simulink model "HYD21"  (R2018b)
settings: configuration reference "Test_Config" (kept outside this file)
undefined symbols (not defined in the file): EDP_PRESS, ENG_SPD_RPM, FALSE, HI_PRES_THRE, LO_PRES_THRS, TRUE
libraries: simulink x16
(part 1 of 2)
settings Model: DataDictionary=ARJ21_Dic.sldd  Creator=maoqiang.huang  LastModifiedBy=IT

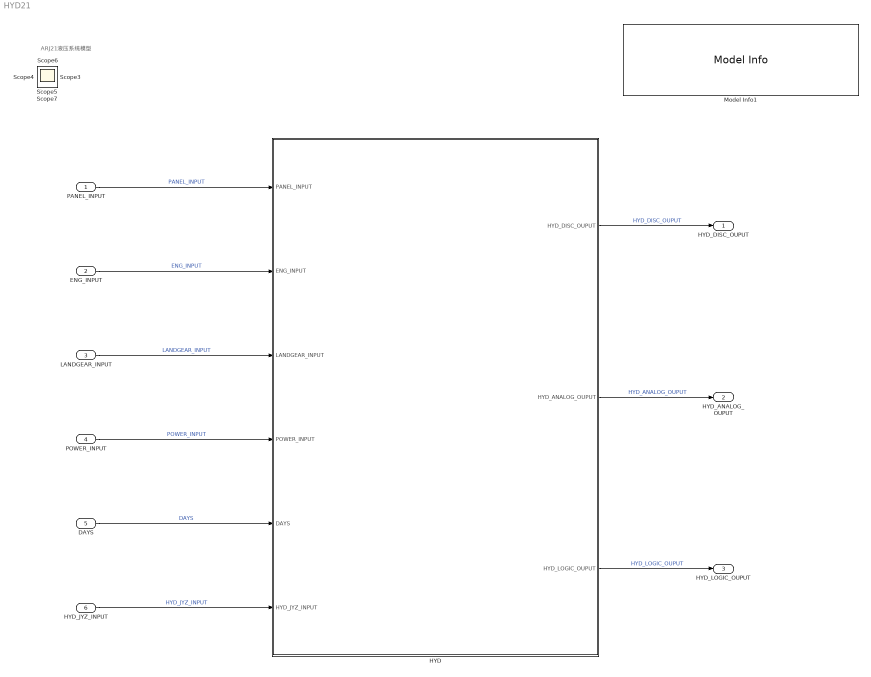
== system HYD21 ==
  note: ARJ21液压系统模型
  PANEL_INPUT : Inport  OutDataTypeStr=Bus: HYD_PANEL_INPUT
  ENG_INPUT : Inport  Port=2  OutDataTypeStr=Bus: HYD_ENG_INPUT
  LANDGEAR_INPUT : Inport  Port=3  OutDataTypeStr=Bus: HYD_LANDGEAR_INPUT
  POWER_INPUT : Inport  Port=4  OutDataTypeStr=Bus: HYD_POWER_INPUT
  DAYS : Inport  Port=5  OutDataTypeStr=uint32
  HYD_JYZ_INPUT : Inport  Port=6  OutDataTypeStr=Bus: HYD_JYZ_INPUT
  HYD : Subsystem
  Model Info1 : simulink/Model-Wide Utilities/Model Info  Frame=on  DisplayStringWithTags=|  HorizontalTextAlignment=Left  LeftAlignmentValue=0.02
      | 创建者：%<Creator>
      | 修改日期：%<ModifiedDate>
      | 模型版本：%<ModelVersion>
  HYD_DISC_OUPUT : Outport  OutDataTypeStr=Bus: HYD_DISC_OUTPUT
  HYD_ANALOG_OUPUT : Outport  Port=2  OutDataTypeStr=Bus: HYD_ANALOG_OUPUT
  HYD_LOGIC_OUPUT : Outport  Port=3  OutDataTypeStr=Bus: HYD_LOGIC_OUPUT
  Scope{,1..7} (8 alike) : Scope
  wires:
  HYD/1(HYD_DISC_OUPUT) -> HYD_DISC_OUPUT/1  "HYD_DISC_OUPUT"
  HYD/2(HYD_ANALOG_OUPUT) -> HYD_ANALOG_OUPUT/1  "HYD_ANALOG_OUPUT"
  PANEL_INPUT/1 -> HYD/1(PANEL_INPUT)  "PANEL_INPUT"
  POWER_INPUT/1 -> HYD/4(POWER_INPUT)  "POWER_INPUT"
  ENG_INPUT/1 -> HYD/2(ENG_INPUT)  "ENG_INPUT"
  LANDGEAR_INPUT/1 -> HYD/3(LANDGEAR_INPUT)  "LANDGEAR_INPUT"
  HYD/3(HYD_LOGIC_OUPUT) -> HYD_LOGIC_OUPUT/1  "HYD_LOGIC_OUPUT"
  DAYS/1 -> HYD/5(DAYS)  "DAYS"
  HYD_JYZ_INPUT/1 -> HYD/6(HYD_JYZ_INPUT)  "HYD_JYZ_INPUT"

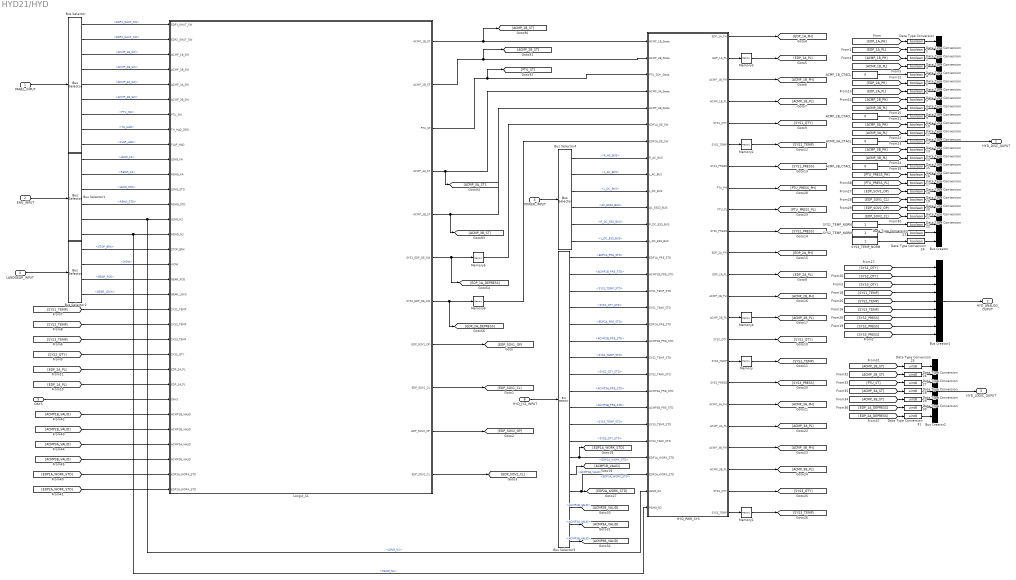
== system HYD21/HYD ==
  PANEL_INPUT : Inport  OutDataTypeStr=Bus: HYD_PANEL_INPUT
  ENG_INPUT : Inport  Port=2  OutDataTypeStr=Bus: HYD_ENG_INPUT
  LANDGEAR_INPUT : Inport  Port=3  OutDataTypeStr=Bus: HYD_LANDGEAR_INPUT
  POWER_INPUT : Inport  Port=4  OutDataTypeStr=Bus: HYD_POWER_INPUT
  DAYS : Inport  Port=5  OutDataTypeStr=uint32
  HYD_JYZ_INPUT : Inport  Port=6  OutDataTypeStr=Bus: HYD_JYZ_INPUT
  ACMP_1B_CTACL : Constant  Value=0
  ACMP_2B_CTACL : Constant  Value=0
  ACMP_3A_CTACL : Constant  Value=0
  ACMP_3B_CTACL : Constant  Value=0
  Bus Creator : BusCreator  Inputs=25  OutDataTypeStr=Bus: HYD_DISC_OUTPUT
  Bus Creator1 : BusCreator  Inputs=9
  Bus Creator2 : BusCreator  Inputs=7
  Bus Selector : BusSelector  OutputSignals=EDP1_SHUT_SW,EDP2_SHUT_SW,ACMP_1B_SW,ACMP_2B_SW,ACMP_3A_SW,ACMP_3B_SW,PTU_SW,TH_HAD,FLAP_HAD
  Bus Selector1 : BusSelector  OutputSignals=LENG_FA,RENG_FA,LENG_STD,RENG_STD,LENG_N2,RENG_N2
  Bus Selector2 : BusSelector  OutputSignals=STOP_BRK,WOW,GEAR_POS,GEAR_LOCK
  Bus Selector3 : BusSelector  OutputSignals=EDP1A_PRE_STD,ACMP1B_PRE_STD,SYS1_TEMP_STD,SYS1_QTY_STD,EDP2A_PRE_STD,ACMP2B_PRE_STD,SYS2_TEMP_STD,SYS2_QTY_STD,ACMP3A_PRE_STD,ACMP3B_PRE_STD,SYS3_TEMP_STD,SYS3_QTY_STD,EDP1A_WORK_STD,ACMP1B_VALID,EDP2A_WORK_STD,ACMP2B_VALID,ACMP3A_VALID,ACMP3B_VALID
  Bus Selector4 : BusSelector  OutputSignals=R_AC_BUS,L_AC_BUS,L_DC_BUS,AC_ESS3_BUS,R_DC_ESS_BUS,L_DC_ESS_BUS
  Data Type Conversion{,1..24} (25 alike) : DataTypeConversion  OutDataTypeStr=boolean
  Data Type Conversion{25..31} (7 alike) : DataTypeConversion  OutDataTypeStr=uint8
  HYD_PWR_SYS : Subsystem
  Locgic_CL : Stateflow chart  TreatAsAtomicUnit=on
  Memory{,1..6} (7 alike) : Memory
  SYS1_TEMP_NORM : Constant
  SYS2_TEMP_NORM : Constant
  SYS3_TEMP_NORM : Constant
  HYD_DISC_OUPUT : Outport  OutDataTypeStr=Bus: HYD_DISC_OUTPUT
  HYD_ANALOG_OUPUT : Outport  Port=2  OutDataTypeStr=Bus: HYD_ANALOG_OUPUT
  HYD_LOGIC_OUPUT : Outport  Port=3  OutDataTypeStr=Bus: HYD_LOGIC_OUPUT
  wires:
  HYD_PWR_SYS/7(SYS1_PRESS) -> [SYS1_PRESS]
  HYD_PWR_SYS/3(ACMP_1B_PH) -> [ACMP_1B_PH]
  Bus Selector1/2 -> Locgic_CL/11(RENG_FA)  "<RENG_FA>"
  [SYS3_TEMP] -> Locgic_CL/22(SYS3_TEMP)
  HYD_PWR_SYS/10(SYS2_PRESS) -> [SYS2_PRESS]
  HYD_PWR_SYS/14(ACMP_2B_PL) -> Memory4/1
  PANEL_INPUT/1 -> Bus Selector/1
  ENG_INPUT/1 -> Bus Selector1/1
  LANDGEAR_INPUT/1 -> Bus Selector2/1
  HYD_PWR_SYS/12(EDP_2A_PL) -> [EDP_2A_PL]
  HYD_PWR_SYS/13(ACMP_2B_PH) -> [ACMP_2B_PH]
  HYD_PWR_SYS/19(ACMP_3A_PL) -> [ACMP_3A_PL]
  Locgic_CL/1(ACMP_1B_ST) -> [ACMP_1B_ST], HYD_PWR_SYS/1(ACMP_1B_State)
  HYD_PWR_SYS/2(EDP_1A_PL) -> Memory3/1
  [EDP_2A_PL] -> Locgic_CL/24(EDP_2A_PL)
  [SYS2_TEMP] -> Locgic_CL/21(SYS2_TEMP)
  Bus Selector1/6 -> HYD_PWR_SYS/29(RENG_N2), Locgic_CL/15(RENG_N2)  "<RENG_N2>"
  HYD_PWR_SYS/20(ACMP_3B_PH) -> [ACMP_3B_PH]
  HYD_PWR_SYS/22(SYS3_QTY) -> [SYS3_QTY]
  Memory6/1 -> HYD_PWR_SYS/7(EDP2A_DE_SW)
  Bus Selector1/5 -> HYD_PWR_SYS/28(LENG_N2), Locgic_CL/14(LENG_N2)  "<LENG_N2>"
  HYD_PWR_SYS/1(EDP_1A_PH) -> [EDP_1A_PH]
  HYD_PWR_SYS/18(ACMP_3A_PH) -> [ACMP_3A_PH]
  HYD_PWR_SYS/15(SYS2_QTY) -> [SYS2_QTY]
  HYD_PWR_SYS/21(ACMP_3B_PL) -> [ACMP_3B_PL]
  Bus Selector1/3 -> Locgic_CL/12(LENG_STD)  "<LENG_STD>"
  HYD_PWR_SYS/17(SYS3_PRESS) -> [SYS3_PRESS]
  Bus Selector/1 -> Locgic_CL/1(EDP1_SHUT_SW)  "<EDP1_SHUT_SW>"
  Bus Selector/6 -> Locgic_CL/6(ACMP_3B_SW)  "<ACMP_3B_SW>"
  Bus Selector/9 -> Locgic_CL/9(FLAP_HAD)  "<FLAP_HAD>"
  Bus Selector/8 -> Locgic_CL/8(TH_HAD_DEG)  "<TH_HAD>"
  Bus Selector/2 -> Locgic_CL/2(EDP2_SHUT_SW)  "<EDP2_SHUT_SW>"
  Bus Selector/5 -> Locgic_CL/5(ACMP_3A_SW)  "<ACMP_3A_SW>"
  Bus Selector/3 -> Locgic_CL/3(ACMP_1B_SW)  "<ACMP_1B_SW>"
  Bus Selector/7 -> Locgic_CL/7(PTU_SW)  "<PTU_SW>"
  Bus Selector/4 -> Locgic_CL/4(ACMP_2B_SW)  "<ACMP_2B_SW>"
  [SYS2_QTY] -> Locgic_CL/23(SYS2_QTY)
  Bus Selector2/1 -> Locgic_CL/16(STOP_BRK)  "<STOP_BRK>"
  Bus Selector2/2 -> Locgic_CL/17(WOW)  "<WOW>"
  Bus Selector2/3 -> Locgic_CL/18(GEAR_POS)  "<GEAR_POS>"
  Bus Selector2/4 -> Locgic_CL/19(GEAR_LOCK)  "<GEAR_LOCK>"
  POWER_INPUT/1 -> Bus Selector4/1
  [SYS1_TEMP] -> Locgic_CL/20(SYS1_TEMP)
  Locgic_CL/8(EDP_SOV1_OP) -> [EDP_SOV1_OP]
  Data Type Conversion11/1 -> Bus Creator/12
  Data Type Conversion12/1 -> Bus Creator/13
  Data Type Conversion3/1 -> Bus Creator/4
  [EDP_1A_PH] -> Data Type Conversion/1
  ACMP_1B_CTACL/1 -> Data Type Conversion4/1
  [EDP_SOV2_OP] -> Data Type Conversion20/1
  Data Type Conversion1/1 -> Bus Creator/2
  Data Type Conversion7/1 -> Bus Creator/8
  Data Type Conversion8/1 -> Bus Creator/9
  ACMP_3A_CTACL/1 -> Data Type Conversion12/1
  [ACMP_3B_PL] -> Data Type Conversion14/1
  SYS1_TEMP_NORM/1 -> Data Type Conversion22/1
  Data Type Conversion4/1 -> Bus Creator/5
  Data Type Conversion10/1 -> Bus Creator/11
  Data Type Conversion13/1 -> Bus Creator/14
  Data Type Conversion14/1 -> Bus Creator/15
  [ACMP_2B_PH] -> Data Type Conversion7/1
  [ACMP_3A_PH] -> Data Type Conversion10/1
  [PTU_PRESS_PH] -> Data Type Conversion16/1
  [ACMP_3B_PH] -> Data Type Conversion13/1
  ACMP_3B_CTACL/1 -> Data Type Conversion15/1
  [EDP_SOV2_CL] -> Data Type Conversion21/1
  Data Type Conversion2/1 -> Bus Creator/3
  Data Type Conversion5/1 -> Bus Creator/6
  [EDP_1A_PL] -> Data Type Conversion1/1
  ACMP_2B_CTACL/1 -> Data Type Conversion9/1
  [EDP_2A_PL] -> Data Type Conversion6/1
  [ACMP_1B_PL] -> Data Type Conversion3/1
  [EDP_2A_PH] -> Data Type Conversion5/1
  [ACMP_2B_PL] -> Data Type Conversion8/1
  [ACMP_3A_PL] -> Data Type Conversion11/1
  [EDP_SOV1_CL] -> Data Type Conversion19/1
  SYS3_TEMP_NORM/1 -> Data Type Conversion24/1
  [EDP_SOV1_OP] -> Data Type Conversion18/1
  SYS2_TEMP_NORM/1 -> Data Type Conversion23/1
  Data Type Conversion/1 -> Bus Creator/1
  [ACMP_1B_PH] -> Data Type Conversion2/1
  Data Type Conversion6/1 -> Bus Creator/7
  Data Type Conversion9/1 -> Bus Creator/10
  Data Type Conversion17/1 -> Bus Creator/18
  [SYS2_QTY] -> Bus Creator1/2
  [SYS3_QTY] -> Bus Creator1/3
  Data Type Conversion21/1 -> Bus Creator/22
  [SYS1_TEMP] -> Bus Creator1/4
  [SYS2_PRESS] -> Bus Creator1/8
  [SYS3_PRESS] -> Bus Creator1/9
  Data Type Conversion24/1 -> Bus Creator/25
  Data Type Conversion23/1 -> Bus Creator/24
  [SYS3_TEMP] -> Bus Creator1/6
  Data Type Conversion15/1 -> Bus Creator/16
  Data Type Conversion18/1 -> Bus Creator/19
  Data Type Conversion20/1 -> Bus Creator/21
  Data Type Conversion22/1 -> Bus Creator/23
  [SYS2_TEMP] -> Bus Creator1/5
  Data Type Conversion19/1 -> Bus Creator/20
  [SYS1_PRESS] -> Bus Creator1/7
  Data Type Conversion16/1 -> Bus Creator/17
  [SYS1_QTY] -> Bus Creator1/1
  Bus Selector4/3 -> HYD_PWR_SYS/10(L_DC_BUS)  "<L_DC_BUS>"
  Bus Selector4/5 -> HYD_PWR_SYS/12(R_DC_ESS_BUS)  "<R_DC_ESS_BUS>"
  Bus Selector4/1 -> HYD_PWR_SYS/8(R_AC_BUS)  "<R_AC_BUS>"
  Bus Selector4/6 -> HYD_PWR_SYS/13(L_DC_ESS_BUS)  "<L_DC_ESS_BUS>"
  Bus Selector4/2 -> HYD_PWR_SYS/9(L_AC_BUS)  "<L_AC_BUS>"
  Bus Selector4/4 -> HYD_PWR_SYS/11(AC_ESS3_BUS)  "<AC_ESS3_BUS>"
  Bus Selector1/4 -> Locgic_CL/13(RENG_STD)  "<RENG_STD>"
  HYD_PWR_SYS/23(SYS3_TEMP) -> Memory1/1
  HYD_PWR_SYS/11(EDP_2A_PH) -> [EDP_2A_PH]
  Memory/1 -> [SYS2_TEMP]
  Bus Selector1/1 -> Locgic_CL/10(LENG_FA)  "<LENG_FA>"
  HYD_PWR_SYS/6(SYS1_TEMP) -> Memory2/1
  [EDP_1A_PL] -> Locgic_CL/25(EDP_1A_PL)
  HYD_PWR_SYS/16(SYS2_TEMP) -> Memory/1
  HYD_PWR_SYS/5(SYS1_QTY) -> [SYS1_QTY]
  Locgic_CL/11(EDP_SOV2_CL) -> [EDP_SOV2_CL]
  Memory1/1 -> [SYS3_TEMP]
  Memory2/1 -> [SYS1_TEMP]
  Memory3/1 -> [EDP_1A_PL]
  Memory4/1 -> [ACMP_2B_PL]
  Memory5/1 -> HYD_PWR_SYS/6(EDP1A_DE_SW)
  HYD_PWR_SYS/4(ACMP_1B_PL) -> [ACMP_1B_PL]
  DAYS/1 -> Locgic_CL/26(DAYS)
  Locgic_CL/9(EDP_SOV1_CL) -> [EDP_SOV1_CL]
  Locgic_CL/6(SYS1_EDP_DE_SW) -> [EDP_1A_DEPRESS], Memory5/1
  Locgic_CL/7(SYS2_EDP_DE_SW) -> [EDP_2A_DEPRESS], Memory6/1
  Locgic_CL/3(PTU_ST) -> [PTU_ST], HYD_PWR_SYS/3(PTU_SOV_State)
  Locgic_CL/5(ACMP_3B_ST) -> [ACMP_3B_ST], HYD_PWR_SYS/5(ACMP_3B_State)
  Locgic_CL/4(ACMP_3A_ST) -> [ACMP_3A_ST], HYD_PWR_SYS/4(ACMP_3A_State)
  Locgic_CL/10(EDP_SOV2_OP) -> [EDP_SOV2_OP]
  Locgic_CL/2(ACMP_2B_ST) -> [ACMP_2B_ST], HYD_PWR_SYS/2(ACMP_2B_State)
  Bus Creator1/1 -> HYD_ANALOG_OUPUT/1
  Bus Creator/1 -> HYD_DISC_OUPUT/1
  HYD_PWR_SYS/8(PTU_PH) -> [PTU_PRESS_PH]
  HYD_PWR_SYS/9(PTU_PL) -> [PTU_PRESS_PL]
  [PTU_PRESS_PL] -> Data Type Conversion17/1
  Bus Creator2/1 -> HYD_LOGIC_OUPUT/1
  [ACMP_2B_ST] -> Data Type Conversion26/1
  [ACMP_3B_ST] -> Data Type Conversion29/1
  [ACMP_3A_ST] -> Data Type Conversion28/1
  [PTU_ST] -> Data Type Conversion27/1
  [ACMP_1B_ST] -> Data Type Conversion25/1
  [EDP_2A_DEPRESS] -> Data Type Conversion31/1
  [EDP_1A_DEPRESS] -> Data Type Conversion30/1
  Data Type Conversion25/1 -> Bus Creator2/1
  Data Type Conversion26/1 -> Bus Creator2/2
  Data Type Conversion27/1 -> Bus Creator2/3
  Data Type Conversion28/1 -> Bus Creator2/4
  Data Type Conversion29/1 -> Bus Creator2/5
  Data Type Conversion30/1 -> Bus Creator2/6
  Data Type Conversion31/1 -> Bus Creator2/7
  HYD_JYZ_INPUT/1 -> Bus Selector3/1
  Bus Selector3/1 -> HYD_PWR_SYS/14(EDP1A_PRE_STD)  "<EDP1A_PRE_STD>"
  Bus Selector3/13 -> HYD_PWR_SYS/26(EDP1A_WORK_STD), [EDP1A_WORK_STD]  "<EDP1A_WORK_STD>"
  Bus Selector3/14 -> [ACMP1B_VALID]  "<ACMP1B_VALID>"
  Bus Selector3/16 -> [ACMP2B_VALID]  "<ACMP2B_VALID>"
  [EDP1A_WORK_STD] -> Locgic_CL/31(EDP1A_WORK_STD)
  [EDP2A_WORK_STD] -> Locgic_CL/32(EDP2A_WORK_STD)
  [ACMP1B_VALID] -> Locgic_CL/27(ACMP1B_VALID)
  [ACMP2B_VALID] -> Locgic_CL/28(ACMP2B_VALID)
  Bus Selector3/17 -> [ACMP3A_VALID]  "<ACMP3A_VALID>"
  Bus Selector3/18 -> [ACMP3B_VALID]  "<ACMP3B_VALID>"
  [ACMP3A_VALID] -> Locgic_CL/29(ACMP3A_VALID)
  [ACMP3B_VALID] -> Locgic_CL/30(ACMP3B_VALID)
  Bus Selector3/2 -> HYD_PWR_SYS/15(ACMP1B_PRE_STD)  "<ACMP1B_PRE_STD>"
  Bus Selector3/3 -> HYD_PWR_SYS/16(SYS1_TEMP_STD)  "<SYS1_TEMP_STD>"
  Bus Selector3/4 -> HYD_PWR_SYS/17(SYS1_TANK_STD)  "<SYS1_QTY_STD>"
  Bus Selector3/5 -> HYD_PWR_SYS/18(EDP2A_PRE_STD)  "<EDP2A_PRE_STD>"
  Bus Selector3/6 -> HYD_PWR_SYS/19(ACMP2B_PRE_STD)  "<ACMP2B_PRE_STD>"
  Bus Selector3/7 -> HYD_PWR_SYS/20(SYS2_TEMP_STD)  "<SYS2_TEMP_STD>"
  Bus Selector3/8 -> HYD_PWR_SYS/21(SYS2_TANK_STD)  "<SYS2_QTY_STD>"
  Bus Selector3/9 -> HYD_PWR_SYS/22(ACMP3A_PRE_STD)  "<ACMP3A_PRE_STD>"
  Bus Selector3/10 -> HYD_PWR_SYS/23(ACMP3B_PRE_STD)  "<ACMP3B_PRE_STD>"
  Bus Selector3/11 -> HYD_PWR_SYS/24(SYS3_TEMP_STD)  "<SYS3_TEMP_STD>"
  Bus Selector3/12 -> HYD_PWR_SYS/25(SYS3_TANK_STD)  "<SYS3_QTY_STD>"
  Bus Selector3/15 -> HYD_PWR_SYS/27(EDP2A_WORK_STD), [EDP2A_WORK_STD]  "<EDP2A_WORK_STD>"

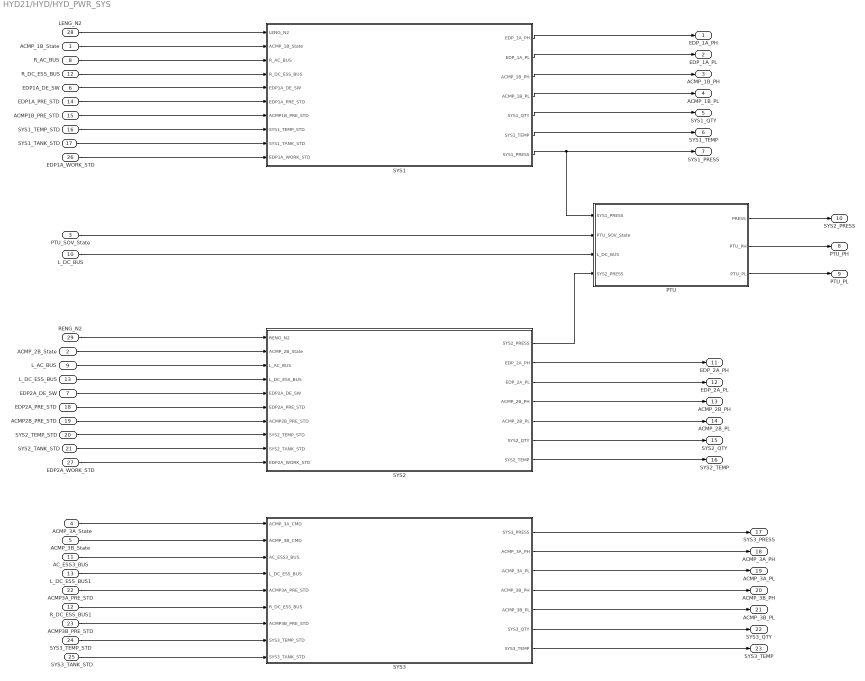
== system HYD21/HYD/HYD_PWR_SYS ==
  ACMP_1B_State : Inport
  ACMP_2B_State : Inport  Port=2
  PTU_SOV_State : Inport  Port=3
  ACMP_3A_State : Inport  Port=4
  ACMP_3B_State : Inport  Port=5
  EDP1A_DE_SW : Inport  Port=6
  EDP2A_DE_SW : Inport  Port=7
  R_AC_BUS : Inport  Port=8
  L_AC_BUS : Inport  Port=9
  L_DC_BUS : Inport  Port=10
  AC_ESS3_BUS : Inport  Port=11
  R_DC_ESS_BUS : Inport  Port=12
  L_DC_ESS_BUS : Inport  Port=13
  EDP1A_PRE_STD : Inport  Port=14
  ACMP1B_PRE_STD : Inport  Port=15
  SYS1_TEMP_STD : Inport  Port=16
  SYS1_TANK_STD : Inport  Port=17
  EDP2A_PRE_STD : Inport  Port=18
  ACMP2B_PRE_STD : Inport  Port=19
  SYS2_TEMP_STD : Inport  Port=20
  SYS2_TANK_STD : Inport  Port=21
  ACMP3A_PRE_STD : Inport  Port=22
  ACMP3B_PRE_STD : Inport  Port=23
  SYS3_TEMP_STD : Inport  Port=24
  SYS3_TANK_STD : Inport  Port=25
  EDP1A_WORK_STD : Inport  Port=26  OutDataTypeStr=uint8
  EDP2A_WORK_STD : Inport  Port=27  OutDataTypeStr=uint8
  LENG_N2 : Inport  Port=28
  RENG_N2 : Inport  Port=29
  L_DC_ESS_BUS1 : InportShadow  Port=13
  PTU : Subsystem
  R_DC_ESS_BUS1 : InportShadow  Port=12
  SYS1 : Subsystem
  SYS2 : Subsystem
  SYS3 : Subsystem
  EDP_1A_PH : Outport
  EDP_1A_PL : Outport  Port=2
  ACMP_1B_PH : Outport  Port=3
  ACMP_1B_PL : Outport  Port=4
  SYS1_QTY : Outport  Port=5
  SYS1_TEMP : Outport  Port=6
  SYS1_PRESS : Outport  Port=7
  PTU_PH : Outport  Port=8
  PTU_PL : Outport  Port=9
  SYS2_PRESS : Outport  Port=10
  EDP_2A_PH : Outport  Port=11
  EDP_2A_PL : Outport  Port=12
  ACMP_2B_PH : Outport  Port=13
  ACMP_2B_PL : Outport  Port=14
  SYS2_QTY : Outport  Port=15
  SYS2_TEMP : Outport  Port=16
  SYS3_PRESS : Outport  Port=17
  ACMP_3A_PH : Outport  Port=18
  ACMP_3A_PL : Outport  Port=19
  ACMP_3B_PH : Outport  Port=20
  ACMP_3B_PL : Outport  Port=21
  SYS3_QTY : Outport  Port=22
  SYS3_TEMP : Outport  Port=23
  wires:
  SYS1/6(SYS1_TEMP) -> SYS1_TEMP/1
  SYS1/3(ACMP_1B_PH) -> ACMP_1B_PH/1
  SYS2/4(ACMP_2B_PH) -> ACMP_2B_PH/1
  SYS2/3(EDP_2A_PL) -> EDP_2A_PL/1
  SYS1/1(EDP_1A_PH) -> EDP_1A_PH/1
  SYS1/2(EDP_1A_PL) -> EDP_1A_PL/1
  SYS1/4(ACMP_1B_PL) -> ACMP_1B_PL/1
  SYS1/5(SYS1_QTY) -> SYS1_QTY/1
  SYS2/2(EDP_2A_PH) -> EDP_2A_PH/1
  SYS2/7(SYS2_TEMP) -> SYS2_TEMP/1
  SYS3/1(SYS3_PRESS) -> SYS3_PRESS/1
  SYS3/7(SYS3_TEMP) -> SYS3_TEMP/1
  SYS2/5(ACMP_2B_PL) -> ACMP_2B_PL/1
  SYS3/4(ACMP_3B_PH) -> ACMP_3B_PH/1
  SYS3/6(SYS3_QTY) -> SYS3_QTY/1
  SYS3/2(ACMP_3A_PH) -> ACMP_3A_PH/1
  SYS2/6(SYS2_QTY) -> SYS2_QTY/1
  SYS3/3(ACMP_3A_PL) -> ACMP_3A_PL/1
  SYS3/5(ACMP_3B_PL) -> ACMP_3B_PL/1
  SYS1/7(SYS1_PRESS) -> SYS1_PRESS/1, PTU/1(SYS1_PRESS)
  LENG_N2/1 -> SYS1/1(LENG_N2)
  ACMP_1B_State/1 -> SYS1/2(ACMP_1B_State)
  EDP1A_DE_SW/1 -> SYS1/5(EDP1A_DE_SW)
  EDP1A_PRE_STD/1 -> SYS1/6(EDP1A_PRE_STD)
  ACMP1B_PRE_STD/1 -> SYS1/7(ACMP1B_PRE_STD)
  SYS1_TEMP_STD/1 -> SYS1/8(SYS1_TEMP_STD)
  SYS1_TANK_STD/1 -> SYS1/9(SYS1_TANK_STD)
  SYS2/1(SYS2_PRESS) -> PTU/4(SYS2_PRESS)
  PTU_SOV_State/1 -> PTU/2(PTU_SOV_State)
  PTU/1(PRESS) -> SYS2_PRESS/1
  L_DC_BUS/1 -> PTU/3(L_DC_BUS)
  ACMP_2B_State/1 -> SYS2/2(ACMP_2B_State)
  RENG_N2/1 -> SYS2/1(RENG_N2)
  L_AC_BUS/1 -> SYS2/3(L_AC_BUS)
  L_DC_ESS_BUS/1 -> SYS2/4(L_DC_ESS_BUS)
  EDP2A_DE_SW/1 -> SYS2/5(EDP2A_DE_SW)
  EDP2A_PRE_STD/1 -> SYS2/6(EDP2A_PRE_STD)
  ACMP2B_PRE_STD/1 -> SYS2/7(ACMP2B_PRE_STD)
  SYS2_TEMP_STD/1 -> SYS2/8(SYS2_TEMP_STD)
  SYS2_TANK_STD/1 -> SYS2/9(SYS2_TANK_STD)
  ACMP_3A_State/1 -> SYS3/1(ACMP_3A_CMD)
  ACMP_3B_State/1 -> SYS3/2(ACMP_3B_CMD)
  L_DC_ESS_BUS1/1 -> SYS3/4(L_DC_ESS_BUS)
  R_DC_ESS_BUS1/1 -> SYS3/6(R_DC_ESS_BUS)
  ACMP3B_PRE_STD/1 -> SYS3/7(ACMP3B_PRE_STD)
  AC_ESS3_BUS/1 -> SYS3/3(AC_ESS3_BUS)
  SYS3_TEMP_STD/1 -> SYS3/8(SYS3_TEMP_STD)
  SYS3_TANK_STD/1 -> SYS3/9(SYS3_TANK_STD)
  ACMP3A_PRE_STD/1 -> SYS3/5(ACMP3A_PRE_STD)
  R_DC_ESS_BUS/1 -> SYS1/4(R_DC_ESS_BUS)
  R_AC_BUS/1 -> SYS1/3(R_AC_BUS)
  PTU/2(PTU_PH) -> PTU_PH/1
  PTU/3(PTU_PL) -> PTU_PL/1
  EDP1A_WORK_STD/1 -> SYS1/10(EDP1A_WORK_STD)
  EDP2A_WORK_STD/1 -> SYS2/10(EDP2A_WORK_STD)

== system HYD21/HYD/HYD_PWR_SYS/PTU ==
  SYS1_PRESS : Inport
  PTU_SOV_State : Inport  Port=2
  L_DC_BUS : Inport  Port=3
  SYS2_PRESS : Inport  Port=4
  Compare To Constant : simulink/Logic and Bit Operations/Compare To Constant  relop=<=  const=1800  OutDataTypeStr=boolean
  HYD2_PRESS_State : Terminator
  Logical Operator : Logic  AllPortsSameDT=off  OutDataTypeStr=boolean
  PRE_SWITCH : Subsystem
  Switch1 : Switch  Criteria=u2 > Threshold  Threshold=LO_PRES_THRS
  PRESS : Outport
  PTU_PH : Outport  Port=2
  PTU_PL : Outport  Port=3
  wires:
  Switch1/1 -> PRE_SWITCH/1(PRE), Compare To Constant/1, PRESS/1
  PTU_SOV_State/1 -> Logical Operator/1
  L_DC_BUS/1 -> Logical Operator/2
  Logical Operator/1 -> Switch1/2
  SYS1_PRESS/1 -> Switch1/1
  SYS2_PRESS/1 -> Switch1/3
  Compare To Constant/1 -> HYD2_PRESS_State/1
  PRE_SWITCH/1(PH) -> PTU_PH/1
  PRE_SWITCH/2(PL) -> PTU_PL/1

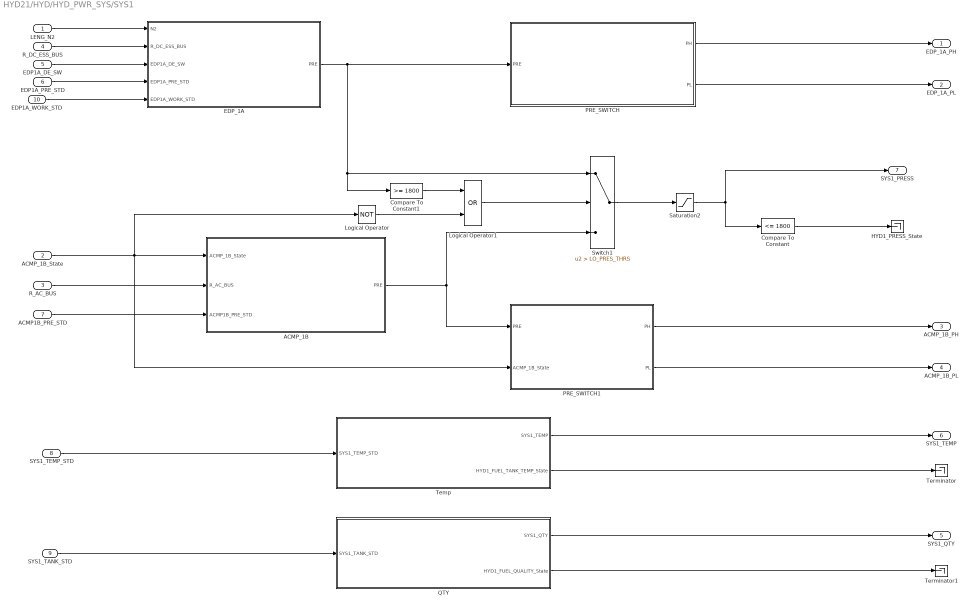
== system HYD21/HYD/HYD_PWR_SYS/SYS1 ==
  LENG_N2 : Inport
  ACMP_1B_State : Inport  Port=2
  R_AC_BUS : Inport  Port=3
  R_DC_ESS_BUS : Inport  Port=4
  EDP1A_DE_SW : Inport  Port=5
  EDP1A_PRE_STD : Inport  Port=6
  ACMP1B_PRE_STD : Inport  Port=7
  SYS1_TEMP_STD : Inport  Port=8
  SYS1_TANK_STD : Inport  Port=9
  EDP1A_WORK_STD : Inport  Port=10  OutDataTypeStr=uint8
  ACMP_1B : Subsystem
  Compare To Constant : simulink/Logic and Bit Operations/Compare To Constant  relop=<=  const=1800  OutDataTypeStr=boolean
  Compare To Constant1 : simulink/Logic and Bit Operations/Compare To Constant  relop=>=  const=1800  OutDataTypeStr=boolean
  EDP_1A : Subsystem
  HYD1_PRESS_State : Terminator
  Logical Operator : Logic  Operator=NOT  AllPortsSameDT=off  OutDataTypeStr=boolean
  Logical Operator1 : Logic  Operator=OR  AllPortsSameDT=off  OutDataTypeStr=boolean
  PRE_SWITCH : Subsystem
  PRE_SWITCH1 : Subsystem
  QTY : Subsystem
  Saturation2 : Saturate  UpperLimit=3000  LowerLimit=0
  Switch1 : Switch  Criteria=u2 > Threshold  Threshold=LO_PRES_THRS
  Temp : Subsystem
  Terminator : Terminator
  Terminator1 : Terminator
  EDP_1A_PH : Outport
  EDP_1A_PL : Outport  Port=2
  ACMP_1B_PH : Outport  Port=3
  ACMP_1B_PL : Outport  Port=4
  SYS1_QTY : Outport  Port=5
  SYS1_TEMP : Outport  Port=6
  SYS1_PRESS : Outport  Port=7
  wires:
  Switch1/1 -> Saturation2/1
  Saturation2/1 -> SYS1_PRESS/1, Compare To Constant/1
  ACMP_1B/1(PRE) -> PRE_SWITCH1/1(PRE), Switch1/3
  PRE_SWITCH/1(PH) -> EDP_1A_PH/1
  PRE_SWITCH/2(PL) -> EDP_1A_PL/1
  EDP_1A/1(PRE) -> Switch1/1, Compare To Constant1/1, PRE_SWITCH/1(PRE)
  PRE_SWITCH1/1(PH) -> ACMP_1B_PH/1
  PRE_SWITCH1/2(PL) -> ACMP_1B_PL/1
  ACMP_1B_State/1 -> PRE_SWITCH1/2(ACMP_1B_State), Logical Operator/1, ACMP_1B/1(ACMP_1B_State)
  Temp/1(SYS1_TEMP) -> SYS1_TEMP/1
  QTY/1(SYS1_QTY) -> SYS1_QTY/1
  LENG_N2/1 -> EDP_1A/1(N2)
  R_DC_ESS_BUS/1 -> EDP_1A/2(R_DC_ESS_BUS)
  EDP1A_DE_SW/1 -> EDP_1A/3(EDP1A_DE_SW)
  EDP1A_PRE_STD/1 -> EDP_1A/4(EDP1A_PRE_STD)
  SYS1_TEMP_STD/1 -> Temp/1(SYS1_TEMP_STD)
  SYS1_TANK_STD/1 -> QTY/1(SYS1_TANK_STD)
  R_AC_BUS/1 -> ACMP_1B/2(R_AC_BUS)
  ACMP1B_PRE_STD/1 -> ACMP_1B/3(ACMP1B_PRE_STD)
  Temp/2("HYD1_FUEL_TANK_TEMP_State ") -> Terminator/1
  QTY/2(HYD1_FUEL_QUALITY_State) -> Terminator1/1
  Compare To Constant/1 -> HYD1_PRESS_State/1
  Logical Operator/1 -> Logical Operator1/2
  Compare To Constant1/1 -> Logical Operator1/1
  Logical Operator1/1 -> Switch1/2
  EDP1A_WORK_STD/1 -> EDP_1A/5(EDP1A_WORK_STD)

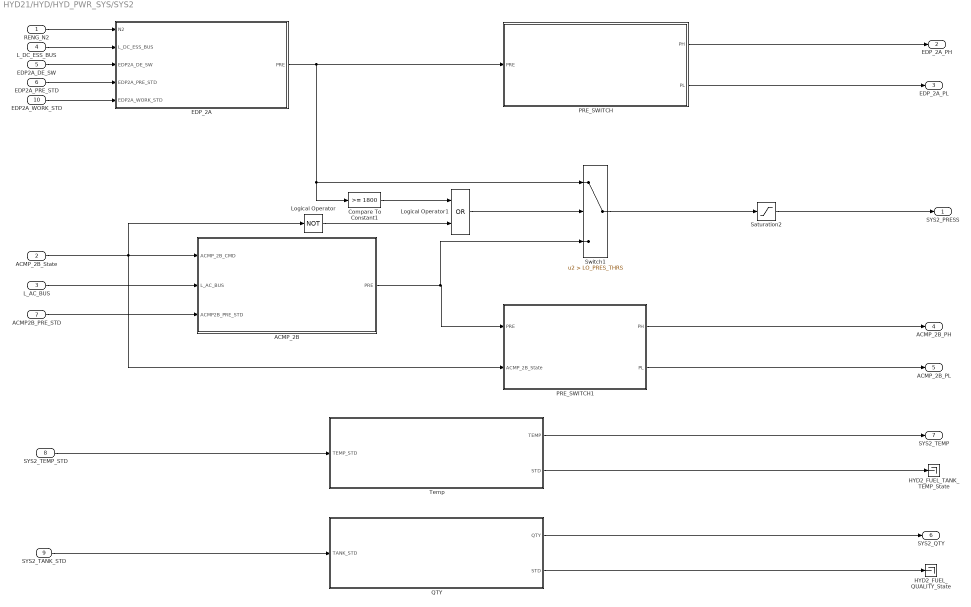
== system HYD21/HYD/HYD_PWR_SYS/SYS2 ==
  RENG_N2 : Inport
  ACMP_2B_State : Inport  Port=2
  L_AC_BUS : Inport  Port=3
  L_DC_ESS_BUS : Inport  Port=4
  EDP2A_DE_SW : Inport  Port=5
  EDP2A_PRE_STD : Inport  Port=6
  ACMP2B_PRE_STD : Inport  Port=7
  SYS2_TEMP_STD : Inport  Port=8
  SYS2_TANK_STD : Inport  Port=9
  EDP2A_WORK_STD : Inport  Port=10  OutDataTypeStr=uint8
  ACMP_2B : Subsystem
  Compare To Constant1 : simulink/Logic and Bit Operations/Compare To Constant  relop=>=  const=1800  OutDataTypeStr=boolean
  EDP_2A : Subsystem
  HYD2_FUEL_QUALITY_State : Terminator
  HYD2_FUEL_TANK_TEMP_State : Terminator
  Logical Operator : Logic  Operator=NOT  AllPortsSameDT=off  OutDataTypeStr=boolean
  Logical Operator1 : Logic  Operator=OR  AllPortsSameDT=off  OutDataTypeStr=boolean
  PRE_SWITCH : Subsystem
  PRE_SWITCH1 : Subsystem
  QTY : Subsystem
  Saturation2 : Saturate  UpperLimit=3000  LowerLimit=0
  Switch1 : Switch  Criteria=u2 > Threshold  Threshold=LO_PRES_THRS
  Temp : Subsystem
  SYS2_PRESS : Outport
  EDP_2A_PH : Outport  Port=2
  EDP_2A_PL : Outport  Port=3
  ACMP_2B_PH : Outport  Port=4
  ACMP_2B_PL : Outport  Port=5
  SYS2_QTY : Outport  Port=6
  SYS2_TEMP : Outport  Port=7
  wires:
  ACMP2B_PRE_STD/1 -> ACMP_2B/3(ACMP2B_PRE_STD)
  L_AC_BUS/1 -> ACMP_2B/2(L_AC_BUS)
  SYS2_TANK_STD/1 -> QTY/1(TANK_STD)
  SYS2_TEMP_STD/1 -> Temp/1(TEMP_STD)
  EDP2A_PRE_STD/1 -> EDP_2A/4(EDP2A_PRE_STD)
  EDP2A_DE_SW/1 -> EDP_2A/3(EDP2A_DE_SW)
  L_DC_ESS_BUS/1 -> EDP_2A/2(L_DC_ESS_BUS)
  RENG_N2/1 -> EDP_2A/1(N2)
  QTY/1(QTY) -> SYS2_QTY/1
  Temp/1(TEMP) -> SYS2_TEMP/1
  ACMP_2B_State/1 -> PRE_SWITCH1/2(ACMP_2B_State), ACMP_2B/1(ACMP_2B_CMD), Logical Operator/1
  PRE_SWITCH1/2(PL) -> ACMP_2B_PL/1
  PRE_SWITCH1/1(PH) -> ACMP_2B_PH/1
  EDP_2A/1(PRE) -> Switch1/1, Compare To Constant1/1, PRE_SWITCH/1(PRE)
  PRE_SWITCH/2(PL) -> EDP_2A_PL/1
  PRE_SWITCH/1(PH) -> EDP_2A_PH/1
  ACMP_2B/1(PRE) -> PRE_SWITCH1/1(PRE), Switch1/3
  Saturation2/1 -> SYS2_PRESS/1
  Switch1/1 -> Saturation2/1
  Temp/2(STD) -> HYD2_FUEL_TANK_TEMP_State/1
  QTY/2(STD) -> HYD2_FUEL_QUALITY_State/1
  Compare To Constant1/1 -> Logical Operator1/1
  Logical Operator/1 -> Logical Operator1/2
  Logical Operator1/1 -> Switch1/2
  EDP2A_WORK_STD/1 -> EDP_2A/5(EDP2A_WORK_STD)

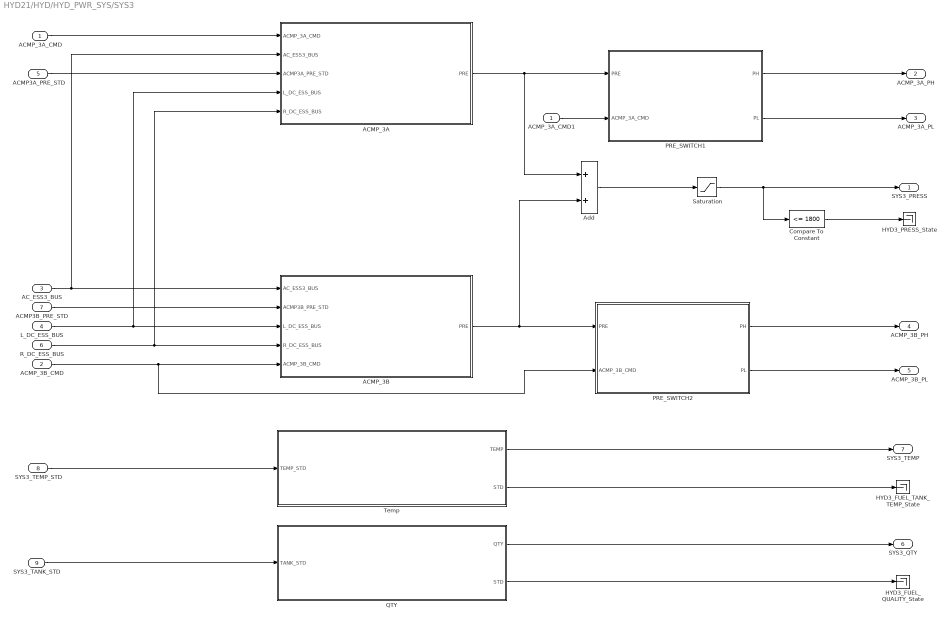
== system HYD21/HYD/HYD_PWR_SYS/SYS3 ==
  ACMP_3A_CMD : Inport
  ACMP_3B_CMD : Inport  Port=2
  AC_ESS3_BUS : Inport  Port=3
  L_DC_ESS_BUS : Inport  Port=4
  ACMP3A_PRE_STD : Inport  Port=5
  R_DC_ESS_BUS : Inport  Port=6
  ACMP3B_PRE_STD : Inport  Port=7
  SYS3_TEMP_STD : Inport  Port=8
  SYS3_TANK_STD : Inport  Port=9
  ACMP_3A : Subsystem
  ACMP_3A_CMD1 : InportShadow
  ACMP_3B : Subsystem
  Add : Sum
  Compare To Constant : simulink/Logic and Bit Operations/Compare To Constant  relop=<=  const=1800  OutDataTypeStr=boolean
  HYD3_FUEL_QUALITY_State : Terminator
  HYD3_FUEL_TANK_TEMP_State : Terminator
  HYD3_PRESS_State : Terminator
  PRE_SWITCH1 : Subsystem
  PRE_SWITCH2 : Subsystem
  QTY : Subsystem
  Saturation : Saturate  UpperLimit=3000  LowerLimit=2800
  Temp : Subsystem
  SYS3_PRESS : Outport
  ACMP_3A_PH : Outport  Port=2
  ACMP_3A_PL : Outport  Port=3
  ACMP_3B_PH : Outport  Port=4
  ACMP_3B_PL : Outport  Port=5
  SYS3_QTY : Outport  Port=6
  SYS3_TEMP : Outport  Port=7
  wires:
  Temp/1(TEMP) -> SYS3_TEMP/1
  QTY/1(QTY) -> SYS3_QTY/1
  SYS3_TANK_STD/1 -> QTY/1(TANK_STD)
  SYS3_TEMP_STD/1 -> Temp/1(TEMP_STD)
  ACMP_3B_CMD/1 -> PRE_SWITCH2/2(ACMP_3B_CMD), ACMP_3B/5(ACMP_3B_CMD)
  AC_ESS3_BUS/1 -> ACMP_3A/2(AC_ESS3_BUS), ACMP_3B/1(AC_ESS3_BUS)
  R_DC_ESS_BUS/1 -> ACMP_3A/5(R_DC_ESS_BUS), ACMP_3B/4(R_DC_ESS_BUS)
  L_DC_ESS_BUS/1 -> ACMP_3A/4(L_DC_ESS_BUS), ACMP_3B/3(L_DC_ESS_BUS)
  ACMP3B_PRE_STD/1 -> ACMP_3B/2(ACMP3B_PRE_STD)
  ACMP_3A_CMD/1 -> ACMP_3A/1(ACMP_3A_CMD)
  ACMP_3B/1(PRE) -> Add/2, PRE_SWITCH2/1(PRE)
  ACMP_3A/1(PRE) -> Add/1, PRE_SWITCH1/1(PRE)
  PRE_SWITCH1/1(PH) -> ACMP_3A_PH/1
  PRE_SWITCH1/2(PL) -> ACMP_3A_PL/1
  PRE_SWITCH2/1(PH) -> ACMP_3B_PH/1
  PRE_SWITCH2/2(PL) -> ACMP_3B_PL/1
  Add/1 -> Saturation/1
  Saturation/1 -> Compare To Constant/1, SYS3_PRESS/1
  ACMP3A_PRE_STD/1 -> ACMP_3A/3(ACMP3A_PRE_STD)
  Compare To Constant/1 -> HYD3_PRESS_State/1
  QTY/2(STD) -> HYD3_FUEL_QUALITY_State/1
  Temp/2(STD) -> HYD3_FUEL_TANK_TEMP_State/1
  ACMP_3A_CMD1/1 -> PRE_SWITCH1/2(ACMP_3A_CMD)

== system HYD21/HYD/HYD_PWR_SYS/PTU/PRE_SWITCH ==
  PRE : Inport
  Constant : Constant  Value=TRUE
  Constant1 : Constant  Value=FALSE
  Constant2 : Constant  Value=TRUE
  Switch : Switch  Criteria=u2 > Threshold  Threshold=HI_PRES_THRE  ZeroCross=off
  Switch1 : Switch  Criteria=u2 > Threshold  Threshold=LO_PRES_THRS
  PH : Outport
  PL : Outport  Port=2
  wires:
  Constant2/1 -> Switch1/3
  Switch1/1 -> PL/1
  Switch/1 -> PH/1
  Constant/1 -> Switch/1
  Constant1/1 -> Switch/3, Switch1/1
  PRE/1 -> Switch/2, Switch1/2

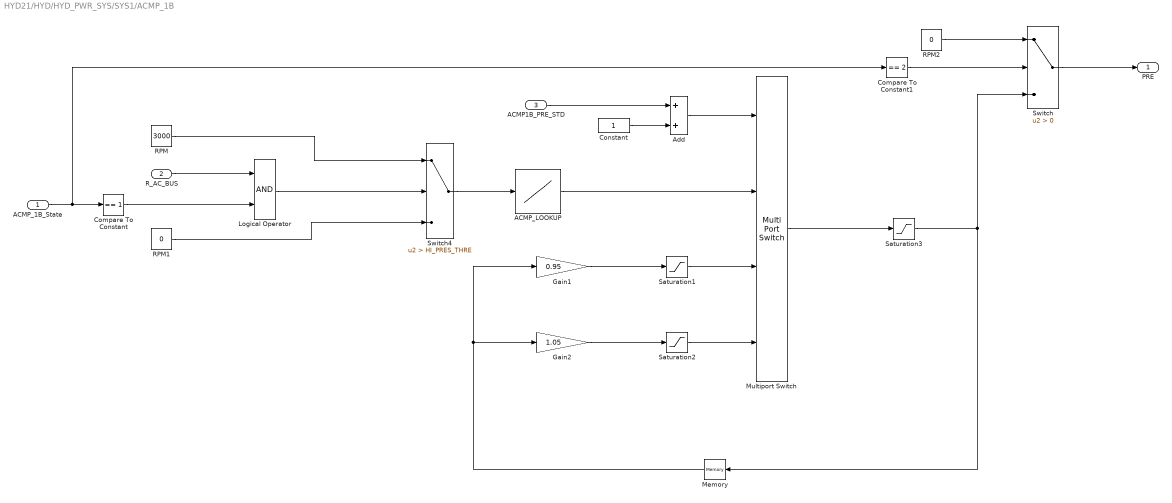
== system HYD21/HYD/HYD_PWR_SYS/SYS1/ACMP_1B ==
  ACMP_1B_State : Inport
  R_AC_BUS : Inport  Port=2
  ACMP1B_PRE_STD : Inport  Port=3
  ACMP_LOOKUP : Lookup_n-D  NumberOfTableDimensions=1  BreakpointsForDimension1=ENG_SPD_RPM  Table=EDP_PRESS  InternalRulePriority=Speed  RndMeth=Simplest  InputSameDT=on
  Add : Sum
  Compare To Constant : simulink/Logic and Bit Operations/Compare To Constant  relop===  const=1  OutDataTypeStr=boolean
  Compare To Constant1 : simulink/Logic and Bit Operations/Compare To Constant  relop===  const=2  OutDataTypeStr=boolean
  Constant : Constant
  Gain1 : Gain  Gain=0.95
  Gain2 : Gain  Gain=1.05
  Logical Operator : Logic  AllPortsSameDT=off  OutDataTypeStr=boolean
  Memory : Memory
  Multiport Switch : MultiPortSwitch  DiagnosticForDefault=None
  RPM : Constant  Value=3000
  RPM1 : Constant  Value=0
  RPM2 : Constant  Value=0
  Saturation1 : Saturate  UpperLimit=3000  LowerLimit=800
  Saturation2 : Saturate  UpperLimit=3500  LowerLimit=3000
  Saturation3 : Saturate  UpperLimit=3000  LowerLimit=0
  Switch : Switch  Criteria=u2 > Threshold
  Switch4 : Switch  Criteria=u2 > Threshold  Threshold=HI_PRES_THRE  ZeroCross=off
  PRE : Outport
  wires:
  Switch4/1 -> ACMP_LOOKUP/1
  RPM/1 -> Switch4/1
  RPM1/1 -> Switch4/3
  R_AC_BUS/1 -> Logical Operator/1
  Logical Operator/1 -> Switch4/2
  Multiport Switch/1 -> Saturation3/1
  Gain1/1 -> Saturation1/1
  Saturation1/1 -> Multiport Switch/3
  Saturation2/1 -> Multiport Switch/4
  Gain2/1 -> Saturation2/1
  Memory/1 -> Gain2/1, Gain1/1
  ACMP_LOOKUP/1 -> Multiport Switch/2
  Saturation3/1 -> Switch/3, Memory/1
  Constant/1 -> Add/2
  ACMP1B_PRE_STD/1 -> Add/1
  Add/1 -> Multiport Switch/1
  Compare To Constant/1 -> Logical Operator/2
  ACMP_1B_State/1 -> Compare To Constant1/1, Compare To Constant/1
  Switch/1 -> PRE/1
  Compare To Constant1/1 -> Switch/2
  RPM2/1 -> Switch/1

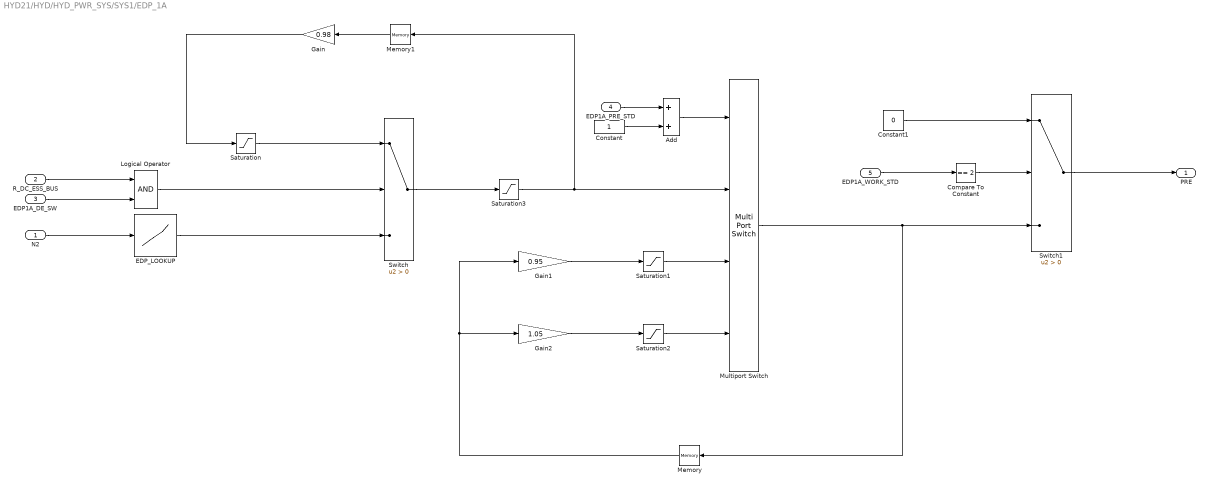
== system HYD21/HYD/HYD_PWR_SYS/SYS1/EDP_1A ==
  N2 : Inport
  R_DC_ESS_BUS : Inport  Port=2
  EDP1A_DE_SW : Inport  Port=3
  EDP1A_PRE_STD : Inport  Port=4
  EDP1A_WORK_STD : Inport  Port=5  OutDataTypeStr=uint8
  Add : Sum
  Compare To Constant : simulink/Logic and Bit Operations/Compare To Constant  relop===  const=2  OutDataTypeStr=boolean
  Constant : Constant
  Constant1 : Constant  Value=0
  EDP_LOOKUP : Lookup_n-D  NumberOfTableDimensions=1  BreakpointsForDimension1=[0 15 20 25 30 35 40 45 50 55 60 65 70 75 80 85 90 95 100]  Table=[0 2000 2200 2400 2600 2800 3000 3000 3000 3000 3000 3000 3000 3000 3000 3000 3000 3000 3000]  InternalRulePriority=Speed  RndMeth=Simplest  InputSameDT=on
  Gain : Gain  Gain=0.98
  Gain1 : Gain  Gain=0.95
  Gain2 : Gain  Gain=1.05
  Logical Operator : Logic  AllPortsSameDT=off  OutDataTypeStr=boolean
  Memory : Memory
  Memory1 : Memory
  Multiport Switch : MultiPortSwitch  DiagnosticForDefault=None
  Saturation : Saturate  UpperLimit=3000  LowerLimit=2000
  Saturation1 : Saturate  UpperLimit=3000  LowerLimit=800
  Saturation2 : Saturate  UpperLimit=3500  LowerLimit=3000
  Saturation3 : Saturate  UpperLimit=3000  LowerLimit=0
  Switch : Switch  Criteria=u2 > Threshold
  Switch1 : Switch  Criteria=u2 > Threshold
  PRE : Outport
  wires:
  N2/1 -> EDP_LOOKUP/1
  Switch/1 -> Saturation3/1
  EDP_LOOKUP/1 -> Switch/3
  R_DC_ESS_BUS/1 -> Logical Operator/1
  EDP1A_DE_SW/1 -> Logical Operator/2
  Logical Operator/1 -> Switch/2
  Gain/1 -> Saturation/1
  Saturation/1 -> Switch/1
  Multiport Switch/1 -> Memory/1, Switch1/3
  Gain1/1 -> Saturation1/1
  Saturation1/1 -> Multiport Switch/3
  Saturation2/1 -> Multiport Switch/4
  Gain2/1 -> Saturation2/1
  Memory/1 -> Gain2/1, Gain1/1
  Memory1/1 -> Gain/1
  Saturation3/1 -> Memory1/1, Multiport Switch/2
  Add/1 -> Multiport Switch/1
  Constant/1 -> Add/2
  EDP1A_PRE_STD/1 -> Add/1
  Constant1/1 -> Switch1/1
  Switch1/1 -> PRE/1
  Compare To Constant/1 -> Switch1/2
  EDP1A_WORK_STD/1 -> Compare To Constant/1

== system HYD21/HYD/HYD_PWR_SYS/SYS1/PRE_SWITCH ==
  PRE : Inport
  Constant : Constant  Value=TRUE
  Constant1 : Constant  Value=FALSE
  Constant2 : Constant  Value=TRUE
  Switch : Switch  Criteria=u2 > Threshold  Threshold=HI_PRES_THRE  ZeroCross=off
  Switch1 : Switch  Criteria=u2 > Threshold  Threshold=LO_PRES_THRS
  PH : Outport
  PL : Outport  Port=2
  wires:
  Constant2/1 -> Switch1/3
  Switch1/1 -> PL/1
  Switch/1 -> PH/1
  Constant/1 -> Switch/1
  Constant1/1 -> Switch/3, Switch1/1
  PRE/1 -> Switch/2, Switch1/2

== system HYD21/HYD/HYD_PWR_SYS/SYS1/PRE_SWITCH1 ==
  PRE : Inport
  ACMP_1B_State : Inport  Port=2
  Constant : Constant  Value=TRUE
  Constant1 : Constant  Value=FALSE
  Constant2 : Constant  Value=TRUE
  Logical Operator : Logic  AllPortsSameDT=off  OutDataTypeStr=boolean
  Switch : Switch  Criteria=u2 > Threshold  Threshold=HI_PRES_THRE  ZeroCross=off
  Switch1 : Switch  Criteria=u2 > Threshold  Threshold=LO_PRES_THRS
  PH : Outport
  PL : Outport  Port=2
  wires:
  Constant/1 -> Switch/1
  Switch/1 -> PH/1
  Switch1/1 -> PL/1
  PRE/1 -> Switch/2, Switch1/2
  ACMP_1B_State/1 -> Logical Operator/2
  Constant1/1 -> Switch/3, Switch1/1
  Constant2/1 -> Logical Operator/1
  Logical Operator/1 -> Switch1/3

== system HYD21/HYD/HYD_PWR_SYS/SYS1/QTY ==
  SYS1_TANK_STD : Inport
  Constant : Constant  Value=80
  Gain : Gain  Gain=0.97
  Logical Operator : Logic  Operator=NOT  AllPortsSameDT=off  OutDataTypeStr=boolean
  Memory : Memory
  Saturation : Saturate  UpperLimit=100  LowerLimit=10
  Switch : Switch  Criteria=u2 > Threshold
  SYS1_QTY : Outport
  HYD1_FUEL_QUALITY_State : Outport  Port=2
  wires:
  Saturation/1 -> Switch/3
  Gain/1 -> Saturation/1
  Constant/1 -> Switch/1
  SYS1_TANK_STD/1 -> HYD1_FUEL_QUALITY_State/1, Logical Operator/1
  Switch/1 -> Memory/1, SYS1_QTY/1
  Memory/1 -> Gain/1
  Logical Operator/1 -> Switch/2

== system HYD21/HYD/HYD_PWR_SYS/SYS1/Temp ==
  SYS1_TEMP_STD : Inport
  Add : Sum
  Constant : Constant  Value=90
  Constant1 : Constant
  Gain : Gain  Gain=1.05
  Gain1 : Gain  Gain=1.05
  Memory : Memory
  Multiport Switch : MultiPortSwitch  DiagnosticForDefault=None
  Saturation : Saturate  UpperLimit=130  LowerLimit=90
  Saturation1 : Saturate  UpperLimit=180  LowerLimit=100
  SYS1_TEMP : Outport
  "HYD1_FUEL_TANK_TEMP_State " : Outport  Port=2
  wires:
  Constant/1 -> Multiport Switch/2
  Multiport Switch/1 -> Memory/1, SYS1_TEMP/1
  Gain/1 -> Saturation/1
  Saturation/1 -> Multiport Switch/3
  Gain1/1 -> Saturation1/1
  Saturation1/1 -> Multiport Switch/4
  SYS1_TEMP_STD/1 -> Add/1, "HYD1_FUEL_TANK_TEMP_State "/1
  Memory/1 -> Gain1/1, Gain/1
  Constant1/1 -> Add/2
  Add/1 -> Multiport Switch/1

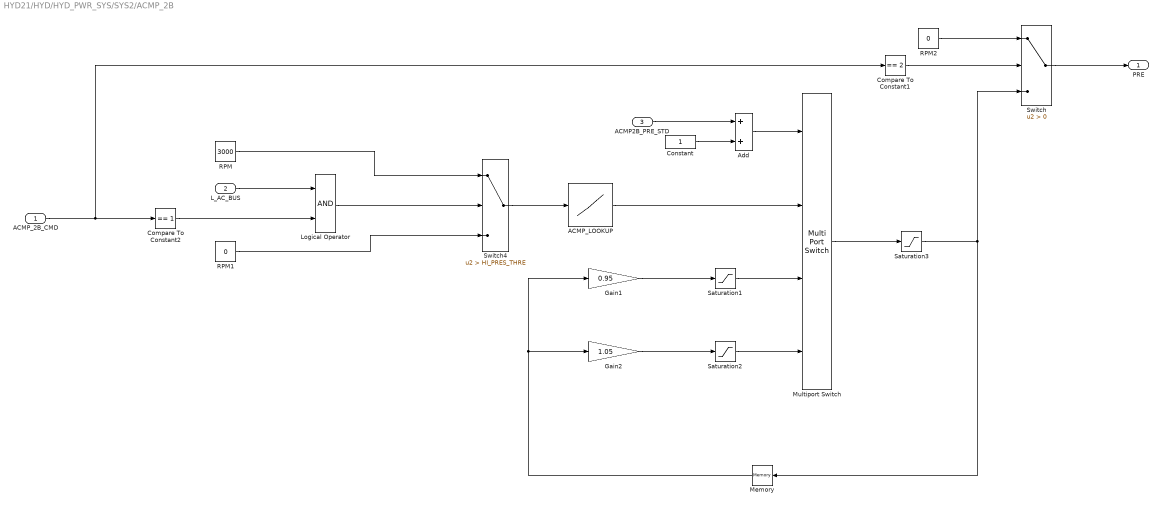
== system HYD21/HYD/HYD_PWR_SYS/SYS2/ACMP_2B ==
  ACMP_2B_CMD : Inport
  L_AC_BUS : Inport  Port=2
  ACMP2B_PRE_STD : Inport  Port=3
  ACMP_LOOKUP : Lookup_n-D  NumberOfTableDimensions=1  BreakpointsForDimension1=ENG_SPD_RPM  Table=EDP_PRESS  InternalRulePriority=Speed  RndMeth=Simplest  InputSameDT=on
  Add : Sum
  Compare To Constant1 : simulink/Logic and Bit Operations/Compare To Constant  relop===  const=2  OutDataTypeStr=boolean
  Compare To Constant2 : simulink/Logic and Bit Operations/Compare To Constant  relop===  const=1  OutDataTypeStr=boolean
  Constant : Constant
  Gain1 : Gain  Gain=0.95
  Gain2 : Gain  Gain=1.05
  Logical Operator : Logic  AllPortsSameDT=off  OutDataTypeStr=boolean
  Memory : Memory
  Multiport Switch : MultiPortSwitch  DiagnosticForDefault=None
  RPM : Constant  Value=3000
  RPM1 : Constant  Value=0
  RPM2 : Constant  Value=0
  Saturation1 : Saturate  UpperLimit=3000  LowerLimit=800
  Saturation2 : Saturate  UpperLimit=3500  LowerLimit=3000
  Saturation3 : Saturate  UpperLimit=3000  LowerLimit=0
  Switch : Switch  Criteria=u2 > Threshold
  Switch4 : Switch  Criteria=u2 > Threshold  Threshold=HI_PRES_THRE  ZeroCross=off
  PRE : Outport
  wires:
  ACMP_LOOKUP/1 -> Multiport Switch/2
  Memory/1 -> Gain1/1, Gain2/1
  Gain2/1 -> Saturation2/1
  Saturation2/1 -> Multiport Switch/4
  Saturation1/1 -> Multiport Switch/3
  Gain1/1 -> Saturation1/1
  Multiport Switch/1 -> Saturation3/1
  Logical Operator/1 -> Switch4/2
  L_AC_BUS/1 -> Logical Operator/1
  RPM1/1 -> Switch4/3
  RPM/1 -> Switch4/1
  Switch4/1 -> ACMP_LOOKUP/1
  Constant/1 -> Add/2
  Add/1 -> Multiport Switch/1
  ACMP2B_PRE_STD/1 -> Add/1
  Compare To Constant1/1 -> Switch/2
  RPM2/1 -> Switch/1
  Switch/1 -> PRE/1
  ACMP_2B_CMD/1 -> Compare To Constant1/1, Compare To Constant2/1
  Saturation3/1 -> Switch/3, Memory/1
  Compare To Constant2/1 -> Logical Operator/2

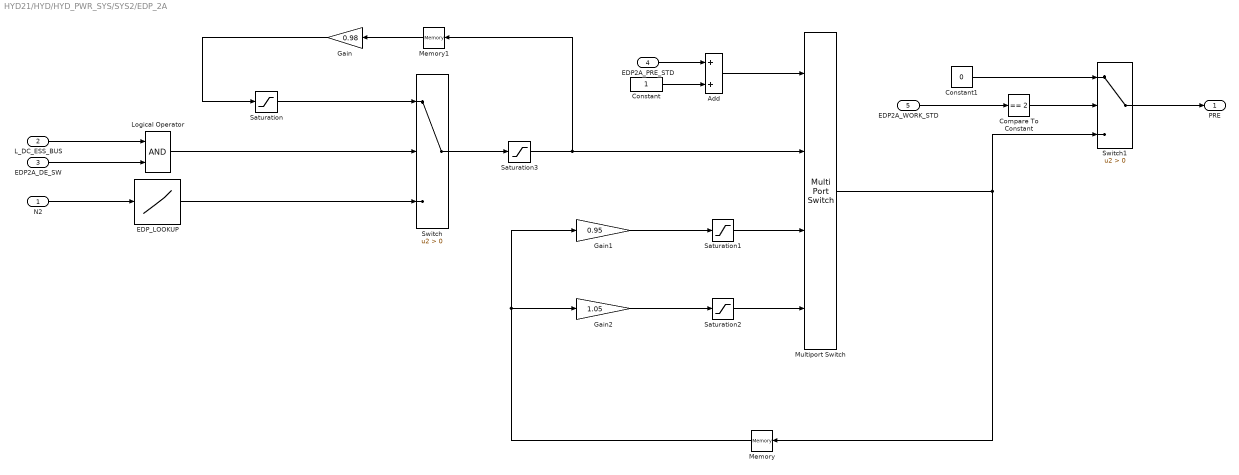
== system HYD21/HYD/HYD_PWR_SYS/SYS2/EDP_2A ==
  N2 : Inport
  L_DC_ESS_BUS : Inport  Port=2
  EDP2A_DE_SW : Inport  Port=3
  EDP2A_PRE_STD : Inport  Port=4
  EDP2A_WORK_STD : Inport  Port=5  OutDataTypeStr=uint8
  Add : Sum
  Compare To Constant : simulink/Logic and Bit Operations/Compare To Constant  relop===  const=2  OutDataTypeStr=boolean
  Constant : Constant
  Constant1 : Constant  Value=0
  EDP_LOOKUP : Lookup_n-D  NumberOfTableDimensions=1  BreakpointsForDimension1=[0 15 20 25 30 35 40 45 50 55 60 65 70 75 80 85 90 95 100]  Table=[0 2000 2200 2400 2600 2800 3000 3000 3000 3000 3000 3000 3000 3000 3000 3000 3000 3000 3000]  InternalRulePriority=Speed  RndMeth=Simplest  InputSameDT=on
  Gain : Gain  Gain=0.98
  Gain1 : Gain  Gain=0.95
  Gain2 : Gain  Gain=1.05
  Logical Operator : Logic  AllPortsSameDT=off  OutDataTypeStr=boolean
  Memory : Memory
  Memory1 : Memory
  Multiport Switch : MultiPortSwitch  DiagnosticForDefault=None
  Saturation : Saturate  UpperLimit=3000  LowerLimit=2000
  Saturation1 : Saturate  UpperLimit=3000  LowerLimit=800
  Saturation2 : Saturate  UpperLimit=3500  LowerLimit=3000
  Saturation3 : Saturate  UpperLimit=3000  LowerLimit=0
  Switch : Switch  Criteria=u2 > Threshold
  Switch1 : Switch  Criteria=u2 > Threshold
  PRE : Outport
  wires:
  Memory/1 -> Gain1/1, Gain2/1
  Gain2/1 -> Saturation2/1
  Saturation2/1 -> Multiport Switch/4
  Saturation1/1 -> Multiport Switch/3
  Gain1/1 -> Saturation1/1
  Multiport Switch/1 -> Switch1/3, Memory/1
  Saturation/1 -> Switch/1
  Gain/1 -> Saturation/1
  EDP2A_DE_SW/1 -> Logical Operator/2
  L_DC_ESS_BUS/1 -> Logical Operator/1
  EDP_LOOKUP/1 -> Switch/3
  Switch/1 -> Saturation3/1
  N2/1 -> EDP_LOOKUP/1
  Memory1/1 -> Gain/1
  Saturation3/1 -> Memory1/1, Multiport Switch/2
  Constant/1 -> Add/2
  Add/1 -> Multiport Switch/1
  EDP2A_PRE_STD/1 -> Add/1
  Logical Operator/1 -> Switch/2
  Switch1/1 -> PRE/1
  Compare To Constant/1 -> Switch1/2
  EDP2A_WORK_STD/1 -> Compare To Constant/1
  Constant1/1 -> Switch1/1

== system HYD21/HYD/HYD_PWR_SYS/SYS2/PRE_SWITCH ==
  PRE : Inport
  Constant : Constant  Value=TRUE
  Constant1 : Constant  Value=FALSE
  Constant2 : Constant  Value=TRUE
  Switch : Switch  Criteria=u2 > Threshold  Threshold=HI_PRES_THRE  ZeroCross=off
  Switch1 : Switch  Criteria=u2 > Threshold  Threshold=LO_PRES_THRS
  PH : Outport
  PL : Outport  Port=2
  wires:
  PRE/1 -> Switch1/2, Switch/2
  Constant1/1 -> Switch1/1, Switch/3
  Constant/1 -> Switch/1
  Switch/1 -> PH/1
  Switch1/1 -> PL/1
  Constant2/1 -> Switch1/3

== system HYD21/HYD/HYD_PWR_SYS/SYS2/PRE_SWITCH1 ==
  PRE : Inport
  ACMP_2B_State : Inport  Port=2
  Constant : Constant  Value=TRUE
  Constant1 : Constant  Value=FALSE
  Constant3 : Constant  Value=TRUE
  Logical Operator : Logic  AllPortsSameDT=off  OutDataTypeStr=boolean
  Switch : Switch  Criteria=u2 > Threshold  Threshold=HI_PRES_THRE  ZeroCross=off
  Switch1 : Switch  Criteria=u2 > Threshold  Threshold=LO_PRES_THRS
  PH : Outport
  PL : Outport  Port=2
  wires:
  Switch1/1 -> PL/1
  Switch/1 -> PH/1
  Constant/1 -> Switch/1
  Constant1/1 -> Switch/3, Switch1/1
  PRE/1 -> Switch/2, Switch1/2
  ACMP_2B_State/1 -> Logical Operator/2
  Constant3/1 -> Logical Operator/1
  Logical Operator/1 -> Switch1/3

== system HYD21/HYD/HYD_PWR_SYS/SYS2/QTY ==
  TANK_STD : Inport
  Constant : Constant  Value=70
  Gain : Gain  Gain=0.97
  Logical Operator : Logic  Operator=NOT  AllPortsSameDT=off  OutDataTypeStr=boolean
  Memory : Memory
  Saturation : Saturate  UpperLimit=100  LowerLimit=8
  Switch : Switch  Criteria=u2 > Threshold
  QTY : Outport
  STD : Outport  Port=2
  wires:
  Switch/1 -> QTY/1, Memory/1
  TANK_STD/1 -> STD/1, Logical Operator/1
  Constant/1 -> Switch/1
  Gain/1 -> Saturation/1
  Saturation/1 -> Switch/3
  Memory/1 -> Gain/1
  Logical Operator/1 -> Switch/2

== system HYD21/HYD/HYD_PWR_SYS/SYS2/Temp ==
  TEMP_STD : Inport
  Add : Sum
  Constant : Constant  Value=88
  Constant1 : Constant
  Gain : Gain  Gain=1.05
  Gain1 : Gain  Gain=1.05
  Memory : Memory
  Multiport Switch : MultiPortSwitch  DiagnosticForDefault=None
  Saturation : Saturate  UpperLimit=130  LowerLimit=60
  Saturation1 : Saturate  UpperLimit=180  LowerLimit=100
  TEMP : Outport
  STD : Outport  Port=2
  wires:
  TEMP_STD/1 -> Add/1, STD/1
  Saturation1/1 -> Multiport Switch/4
  Gain1/1 -> Saturation1/1
  Saturation/1 -> Multiport Switch/3
  Gain/1 -> Saturation/1
  Multiport Switch/1 -> TEMP/1, Memory/1
  Constant/1 -> Multiport Switch/2
  Memory/1 -> Gain/1, Gain1/1
  Constant1/1 -> Add/2
  Add/1 -> Multiport Switch/1

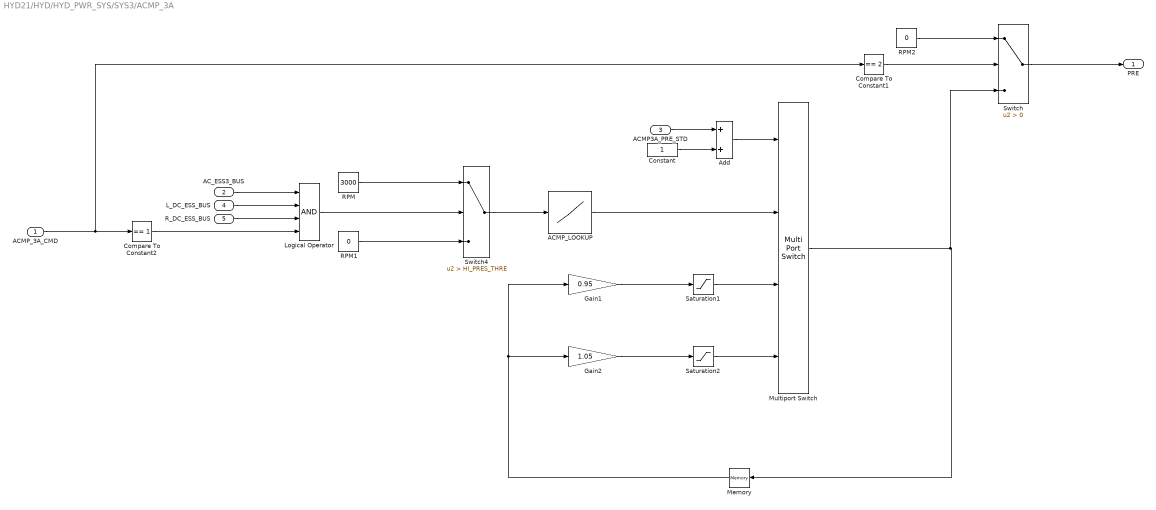
== system HYD21/HYD/HYD_PWR_SYS/SYS3/ACMP_3A ==
  ACMP_3A_CMD : Inport
  AC_ESS3_BUS : Inport  Port=2
  ACMP3A_PRE_STD : Inport  Port=3
  L_DC_ESS_BUS : Inport  Port=4
  R_DC_ESS_BUS : Inport  Port=5
  ACMP_LOOKUP : Lookup_n-D  NumberOfTableDimensions=1  BreakpointsForDimension1=ENG_SPD_RPM  Table=EDP_PRESS  InternalRulePriority=Speed  RndMeth=Simplest  InputSameDT=on
  Add : Sum
  Compare To Constant1 : simulink/Logic and Bit Operations/Compare To Constant  relop===  const=2  OutDataTypeStr=boolean
  Compare To Constant2 : simulink/Logic and Bit Operations/Compare To Constant  relop===  const=1  OutDataTypeStr=boolean
  Constant : Constant
  Gain1 : Gain  Gain=0.95
  Gain2 : Gain  Gain=1.05
  Logical Operator : Logic  Inputs=4  AllPortsSameDT=off  OutDataTypeStr=boolean
  Memory : Memory
  Multiport Switch : MultiPortSwitch  DiagnosticForDefault=None
  RPM : Constant  Value=3000
  RPM1 : Constant  Value=0
  RPM2 : Constant  Value=0
  Saturation1 : Saturate  UpperLimit=3000  LowerLimit=800
  Saturation2 : Saturate  UpperLimit=3500  LowerLimit=3000
  Switch : Switch  Criteria=u2 > Threshold
  Switch4 : Switch  Criteria=u2 > Threshold  Threshold=HI_PRES_THRE  ZeroCross=off
  PRE : Outport
  wires:
  AC_ESS3_BUS/1 -> Logical Operator/1
  L_DC_ESS_BUS/1 -> Logical Operator/2
  R_DC_ESS_BUS/1 -> Logical Operator/3
  Switch4/1 -> ACMP_LOOKUP/1
  RPM/1 -> Switch4/1
  RPM1/1 -> Switch4/3
  Logical Operator/1 -> Switch4/2
  Gain1/1 -> Saturation1/1
  Saturation1/1 -> Multiport Switch/3
  Saturation2/1 -> Multiport Switch/4
  Gain2/1 -> Saturation2/1
  Memory/1 -> Gain2/1, Gain1/1
  ACMP_LOOKUP/1 -> Multiport Switch/2
  Constant/1 -> Add/2
  Add/1 -> Multiport Switch/1
  ACMP3A_PRE_STD/1 -> Add/1
  RPM2/1 -> Switch/1
  Multiport Switch/1 -> Switch/3, Memory/1
  Compare To Constant1/1 -> Switch/2
  Switch/1 -> PRE/1
  ACMP_3A_CMD/1 -> Compare To Constant1/1, Compare To Constant2/1
  Compare To Constant2/1 -> Logical Operator/4

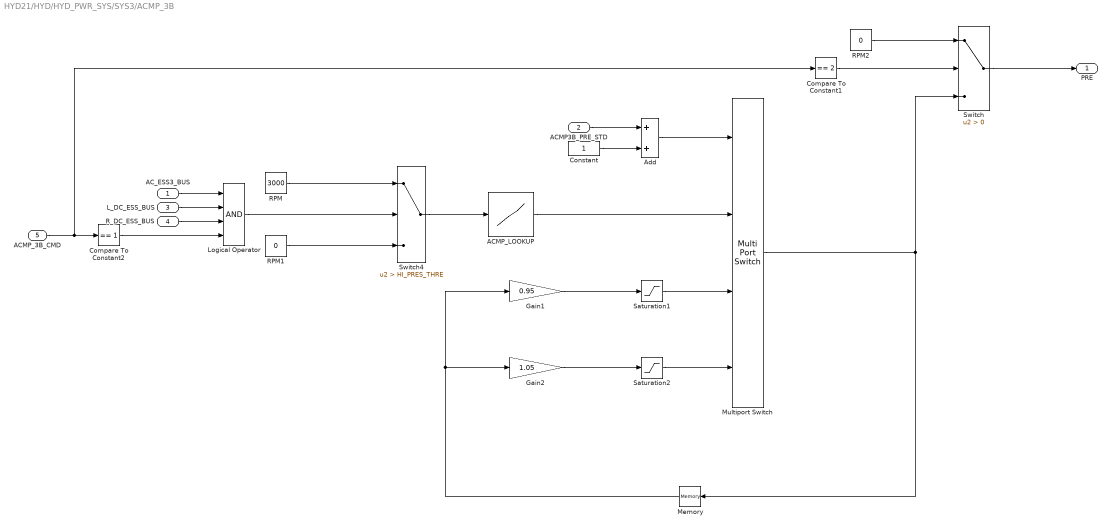
== system HYD21/HYD/HYD_PWR_SYS/SYS3/ACMP_3B ==
  AC_ESS3_BUS : Inport
  ACMP3B_PRE_STD : Inport  Port=2
  L_DC_ESS_BUS : Inport  Port=3
  R_DC_ESS_BUS : Inport  Port=4
  ACMP_3B_CMD : Inport  Port=5
  ACMP_LOOKUP : Lookup_n-D  NumberOfTableDimensions=1  BreakpointsForDimension1=ENG_SPD_RPM  Table=EDP_PRESS  InternalRulePriority=Speed  RndMeth=Simplest  InputSameDT=on
  Add : Sum
  Compare To Constant1 : simulink/Logic and Bit Operations/Compare To Constant  relop===  const=2  OutDataTypeStr=boolean
  Compare To Constant2 : simulink/Logic and Bit Operations/Compare To Constant  relop===  const=1  OutDataTypeStr=boolean
  Constant : Constant
  Gain1 : Gain  Gain=0.95
  Gain2 : Gain  Gain=1.05
  Logical Operator : Logic  Inputs=4  AllPortsSameDT=off  OutDataTypeStr=boolean
  Memory : Memory
  Multiport Switch : MultiPortSwitch  DiagnosticForDefault=None
  RPM : Constant  Value=3000
  RPM1 : Constant  Value=0
  RPM2 : Constant  Value=0
  Saturation1 : Saturate  UpperLimit=3000  LowerLimit=800
  Saturation2 : Saturate  UpperLimit=3500  LowerLimit=3000
  Switch : Switch  Criteria=u2 > Threshold
  Switch4 : Switch  Criteria=u2 > Threshold  Threshold=HI_PRES_THRE  ZeroCross=off
  PRE : Outport
  wires:
  ACMP_LOOKUP/1 -> Multiport Switch/2
  Memory/1 -> Gain1/1, Gain2/1
  Gain2/1 -> Saturation2/1
  Saturation2/1 -> Multiport Switch/4
  Saturation1/1 -> Multiport Switch/3
  Gain1/1 -> Saturation1/1
  Logical Operator/1 -> Switch4/2
  RPM1/1 -> Switch4/3
  RPM/1 -> Switch4/1
  Switch4/1 -> ACMP_LOOKUP/1
  ACMP_3B_CMD/1 -> Compare To Constant1/1, Compare To Constant2/1
  R_DC_ESS_BUS/1 -> Logical Operator/3
  L_DC_ESS_BUS/1 -> Logical Operator/2
  AC_ESS3_BUS/1 -> Logical Operator/1
  Constant/1 -> Add/2
  Add/1 -> Multiport Switch/1
  ACMP3B_PRE_STD/1 -> Add/1
  RPM2/1 -> Switch/1
  Multiport Switch/1 -> Switch/3, Memory/1
  Compare To Constant1/1 -> Switch/2
  Switch/1 -> PRE/1
  Compare To Constant2/1 -> Logical Operator/4

== system HYD21/HYD/HYD_PWR_SYS/SYS3/PRE_SWITCH1 ==
  PRE : Inport
  ACMP_3A_CMD : Inport  Port=2
  Constant : Constant  Value=TRUE
  Constant1 : Constant  Value=FALSE
  Constant2 : Constant  Value=TRUE
  Logical Operator : Logic  AllPortsSameDT=off  OutDataTypeStr=boolean
  Switch : Switch  Criteria=u2 > Threshold  Threshold=HI_PRES_THRE  ZeroCross=off
  Switch1 : Switch  Criteria=u2 > Threshold  Threshold=LO_PRES_THRS
  PH : Outport
  PL : Outport  Port=2
  wires:
  Switch1/1 -> PL/1
  Switch/1 -> PH/1
  Constant/1 -> Switch/1
  Constant1/1 -> Switch/3, Switch1/1
  PRE/1 -> Switch/2, Switch1/2
  ACMP_3A_CMD/1 -> Logical Operator/2
  Constant2/1 -> Logical Operator/1
  Logical Operator/1 -> Switch1/3

== system HYD21/HYD/HYD_PWR_SYS/SYS3/PRE_SWITCH2 ==
  PRE : Inport
  ACMP_3B_CMD : Inport  Port=2
  Constant : Constant  Value=TRUE
  Constant1 : Constant  Value=FALSE
  Constant2 : Constant  Value=TRUE
  Logical Operator : Logic  AllPortsSameDT=off  OutDataTypeStr=boolean
  Switch : Switch  Criteria=u2 > Threshold  Threshold=HI_PRES_THRE  ZeroCross=off
  Switch1 : Switch  Criteria=u2 > Threshold  Threshold=LO_PRES_THRS
  PH : Outport
  PL : Outport  Port=2
  wires:
  PRE/1 -> Switch1/2, Switch/2
  Constant1/1 -> Switch1/1, Switch/3
  Constant/1 -> Switch/1
  Switch/1 -> PH/1
  Switch1/1 -> PL/1
  ACMP_3B_CMD/1 -> Logical Operator/2
  Constant2/1 -> Logical Operator/1
  Logical Operator/1 -> Switch1/3

== system HYD21/HYD/HYD_PWR_SYS/SYS3/QTY ==
  TANK_STD : Inport
  Constant : Constant  Value=84
  Gain : Gain  Gain=0.97
  Logical Operator : Logic  Operator=NOT  AllPortsSameDT=off  OutDataTypeStr=boolean
  Memory : Memory
  Saturation : Saturate  UpperLimit=100  LowerLimit=15
  Switch : Switch  Criteria=u2 > Threshold
  QTY : Outport
  STD : Outport  Port=2
  wires:
  Switch/1 -> QTY/1, Memory/1
  TANK_STD/1 -> STD/1, Logical Operator/1
  Constant/1 -> Switch/1
  Gain/1 -> Saturation/1
  Saturation/1 -> Switch/3
  Memory/1 -> Gain/1
  Logical Operator/1 -> Switch/2

== system HYD21/HYD/HYD_PWR_SYS/SYS3/Temp ==
  TEMP_STD : Inport
  Add : Sum
  Constant : Constant  Value=95
  Constant1 : Constant
  Gain : Gain  Gain=1.05
  Gain1 : Gain  Gain=1.05
  Memory : Memory
  Multiport Switch : MultiPortSwitch  DiagnosticForDefault=None
  Saturation : Saturate  UpperLimit=130  LowerLimit=60
  Saturation1 : Saturate  UpperLimit=180  LowerLimit=100
  TEMP : Outport
  STD : Outport  Port=2
  wires:
  TEMP_STD/1 -> Add/1, STD/1
  Saturation1/1 -> Multiport Switch/4
  Gain1/1 -> Saturation1/1
  Saturation/1 -> Multiport Switch/3
  Gain/1 -> Saturation/1
  Multiport Switch/1 -> TEMP/1, Memory/1
  Constant/1 -> Multiport Switch/2
  Memory/1 -> Gain/1, Gain1/1
  Constant1/1 -> Add/2
  Add/1 -> Multiport Switch/1
